simulink model "RaketenMolell_V1"  (R2021b)
settings: Solver=VariableStepAuto  StartTime=0.0  StopTime=10.0  RelTol=1e-3
values from neighbouring files (symbols this model uses):
  ObjectMass = 3    [RaketeParameter.m]
  PropGain = 10    [RaketeParameter.m]
settings Model: Creator=tim  LastModifiedBy=tim

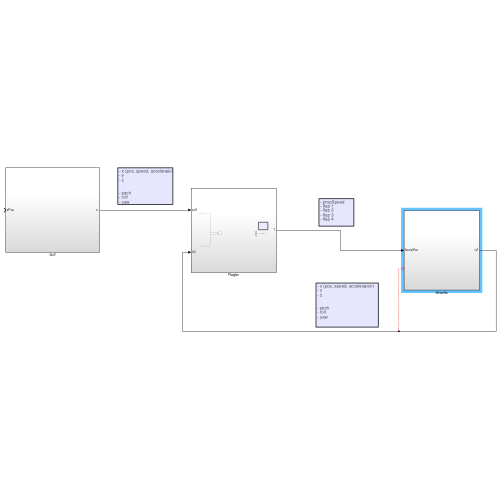
[thumbnail: Simulink's stored preview of the top-level diagram]
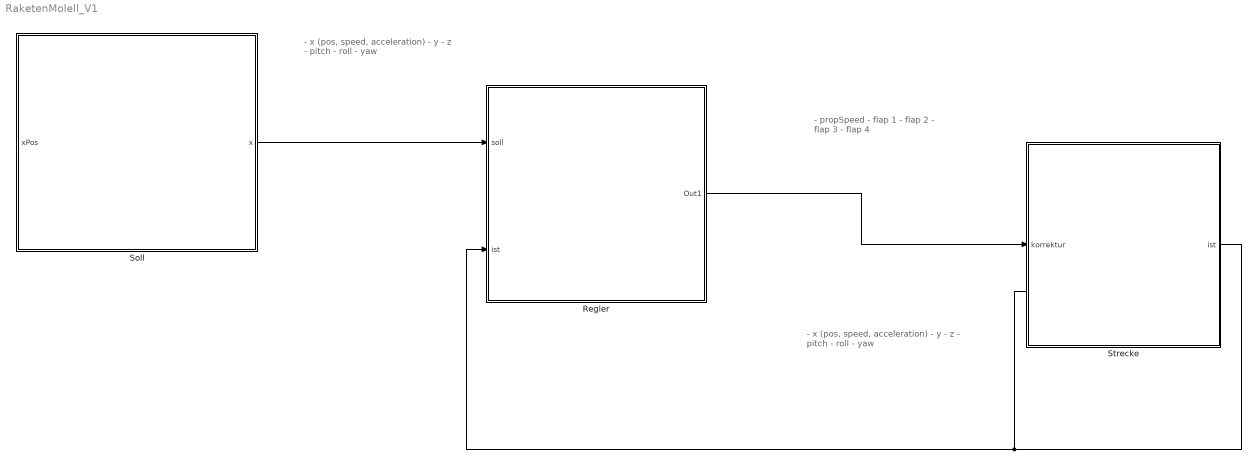
== system RaketenMolell_V1 ==
  note: - x (pos, speed, acceleration)
      | - y
      | - z
      |
      |
      | - pitch
      | - roll
      | - yaw
  note: - propSpeed
      | - flap 1
      | - flap 2
      | - flap 3
      | - flap 4
  note: - x (pos, speed, acceleration)
      | - y
      | - z
      |
      |
      | - pitch
      | - roll
      | - yaw
  Regler : Subsystem
  Soll : Subsystem
  Strecke : Subsystem
  wires:
  Soll/1(x) -> Regler/1(soll)
  Strecke/1(ist) -> Regler/2(ist)
  Regler/1(Out1) -> Strecke/1(korrektur)

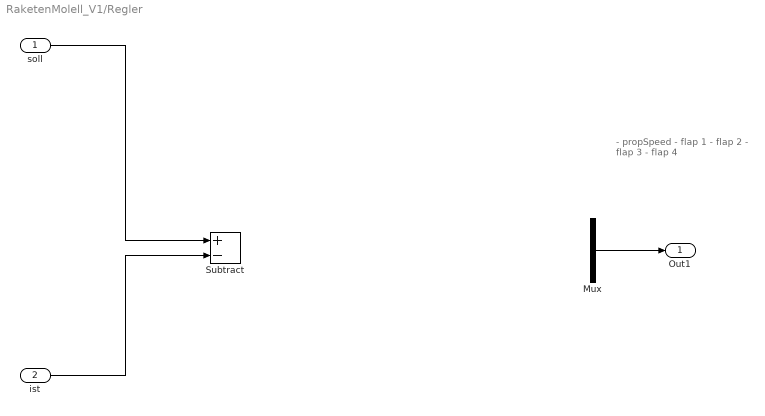
== system RaketenMolell_V1/Regler ==
  note: - propSpeed
      | - flap 1
      | - flap 2
      | - flap 3
      | - flap 4
  soll : Inport
  ist : Inport  Port=2
  Mux : Mux  Inputs=5
  Subtract : Sum  Inputs=+-
  Out1 : Outport
  wires:
  soll/1 -> Subtract/1
  ist/1 -> Subtract/2
  Mux/1 -> Out1/1

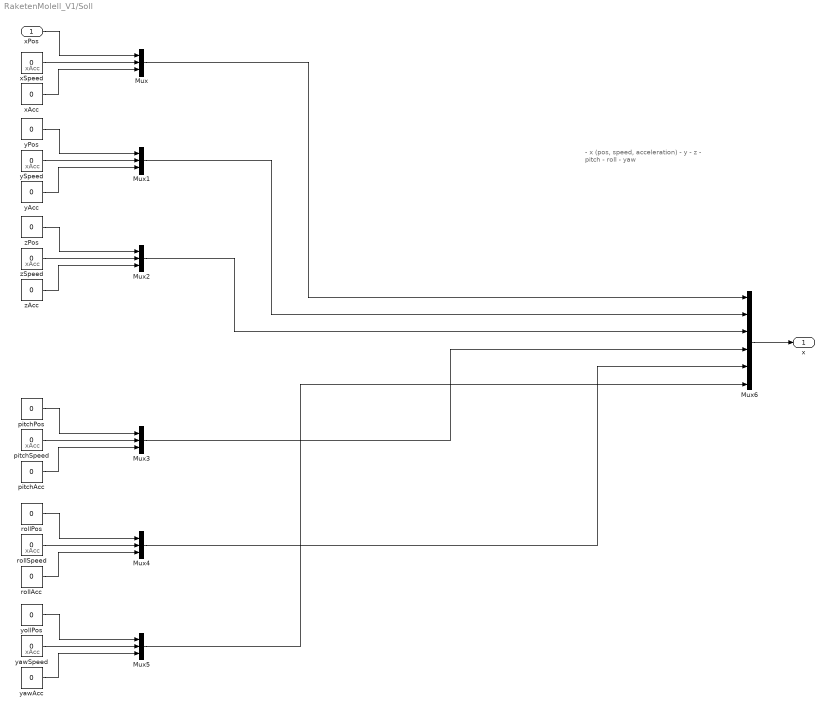
== system RaketenMolell_V1/Soll ==
  note: - x (pos, speed, acceleration)
      | - y
      | - z
      |
      |
      | - pitch
      | - roll
      | - yaw
  note: xAcc
  note: xAcc
  note: xAcc
  note: xAcc
  note: xAcc
  note: xAcc
  xPos : Inport
  Mux{,1..5} (6 alike) : Mux  Inputs=3
  Mux6 : Mux  Inputs=6
  pitchAcc : Constant  Value=0
  pitchPos : Constant  Value=0
  pitchSpeed : Constant  Value=0
  rollAcc : Constant  Value=0
  rollPos : Constant  Value=0
  rollSpeed : Constant  Value=0
  xAcc : Constant  Value=0
  xSpeed : Constant  Value=0
  yAcc : Constant  Value=0
  yPos : Constant  Value=0
  ySpeed : Constant  Value=0
  yawAcc : Constant  Value=0
  yawSpeed : Constant  Value=0
  yollPos : Constant  Value=0
  zAcc : Constant  Value=0
  zPos : Constant  Value=0
  zSpeed : Constant  Value=0
  x : Outport
  wires:
  xPos/1 -> Mux/1
  xSpeed/1 -> Mux/2
  Mux/1 -> Mux6/1
  Mux1/1 -> Mux6/2
  Mux2/1 -> Mux6/3
  xAcc/1 -> Mux/3
  yPos/1 -> Mux1/1
  ySpeed/1 -> Mux1/2
  yAcc/1 -> Mux1/3
  zPos/1 -> Mux2/1
  zSpeed/1 -> Mux2/2
  zAcc/1 -> Mux2/3
  Mux4/1 -> Mux6/5
  rollAcc/1 -> Mux4/3
  Mux5/1 -> Mux6/6
  pitchPos/1 -> Mux3/1
  Mux3/1 -> Mux6/4
  yollPos/1 -> Mux5/1
  yawAcc/1 -> Mux5/3
  yawSpeed/1 -> Mux5/2
  rollPos/1 -> Mux4/1
  rollSpeed/1 -> Mux4/2
  pitchSpeed/1 -> Mux3/2
  pitchAcc/1 -> Mux3/3
  Mux6/1 -> x/1

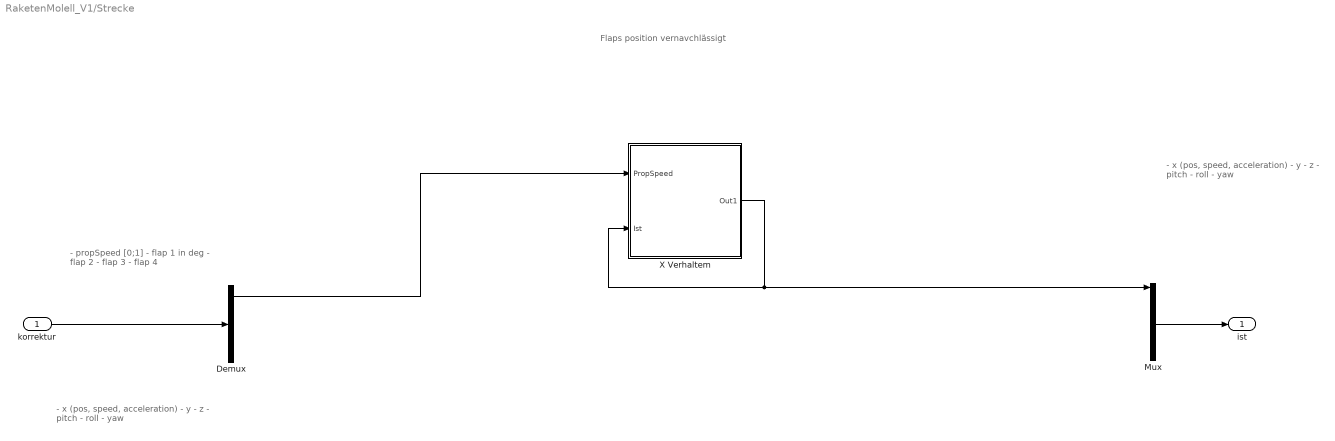
== system RaketenMolell_V1/Strecke ==
  note: Flaps position
      | vernavchlässigt
  note: - propSpeed [0;1]
      | - flap 1          in deg
      | - flap 2
      | - flap 3
      | - flap 4
  note: - x (pos, speed, acceleration)
      | - y
      | - z
      |
      |
      | - pitch
      | - roll
      | - yaw
  note: - x (pos, speed, acceleration)
      | - y
      | - z
      |
      |
      | - pitch
      | - roll
      | - yaw
  korrektur : Inport
  Demux : Demux  Outputs=5
  Mux : Mux  Inputs=6
  X Verhaltem : Subsystem
  ist : Outport
  wires:
  Demux/1 -> X Verhaltem/1(PropSpeed)
  Mux/1 -> ist/1
  X Verhaltem/1(Out1) -> Mux/1, X Verhaltem/2(Ist)
  korrektur/1 -> Demux/1

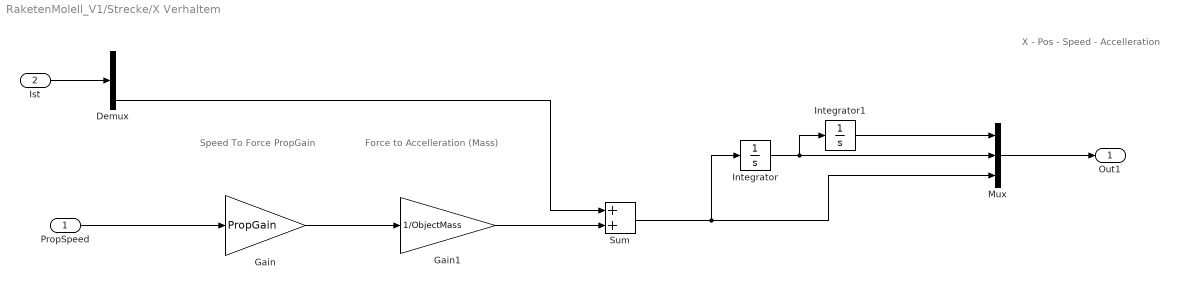
== system RaketenMolell_V1/Strecke/X Verhaltem ==
  note: Speed To Force
      | PropGain
  note: X
      | - Pos
      | - Speed
      | - Accelleration
  note: Force to Accelleration
      | (Mass)
  PropSpeed : Inport
  Ist : Inport  Port=2
  Demux : Demux  Outputs=3
  Gain : Gain  Gain=PropGain
  Gain1 : Gain  Gain=1/ObjectMass
  Integrator : Integrator
  Integrator1 : Integrator
  Mux : Mux  Inputs=3
  Sum : Sum
  Out1 : Outport
  wires:
  Mux/1 -> Out1/1
  PropSpeed/1 -> Gain/1
  Gain/1 -> Gain1/1
  Gain1/1 -> Sum/2
  Ist/1 -> Demux/1
  Demux/3 -> Sum/1
  Sum/1 -> Integrator/1, Mux/3
  Integrator/1 -> Integrator1/1, Mux/2
  Integrator1/1 -> Mux/1
